simulink model "ex6_dvbs_chain"  (R2022a)
settings: Solver=FixedStepAuto  StartTime=0  StopTime=Tsim  RelTol=1e-3
values from neighbouring files (symbols this model uses):
  Rb = 100e3    (= 100000)    [ex6_parameters.m]
  RS_k = 188    [ex6_parameters.m]
  RS_m = 8    [ex6_parameters.m]
  RS_n = 204    [ex6_parameters.m]
  RS_prim_poly = 'X^8+X^4+X^3+X^2+1'    [ex6_parameters.m]
  VIT_cv1 = 171    [ex6_parameters.m]
  VIT_cv2 = 133    [ex6_parameters.m]
  VIT_K = 7    [ex6_parameters.m]
undefined symbols (not defined in the file or in its folder): rsgenpoly
libraries: commsink2 x2, commblkcod2 x2, commcnvcod2 x2, commsequence2 x2, commblkintrlv2 x2, commrandsrc3 x1, commchan3 x1
settings Model: Creator=root  LastModifiedBy=Filippo
settings SolverCC: AlgebraicLoopSolver=TrustRegion
settings DataIOCC: ReturnWorkspaceOutputs=off
settings DebuggingCC: UnconnectedInputMsg=warning  UnconnectedOutputMsg=warning  UnconnectedLineMsg=warning  SFMachineParentedDataDiag=warning  ArithmeticOperatorsInVariantConditions=warning
settings SFSimCC: SimUseLocalCustomCode=off  CustomCodeUndefinedFunction=UseInterfaceOnly
settings RTWCC: RTWUseLocalCustomCode=off
settings CodeAppCC: StateflowObjectComments=on

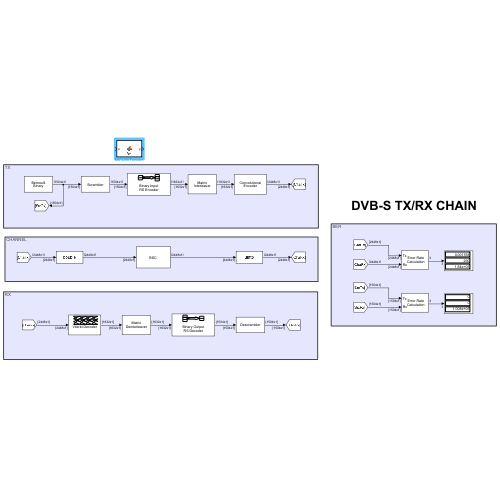
[thumbnail: Simulink's stored preview of the top-level diagram]
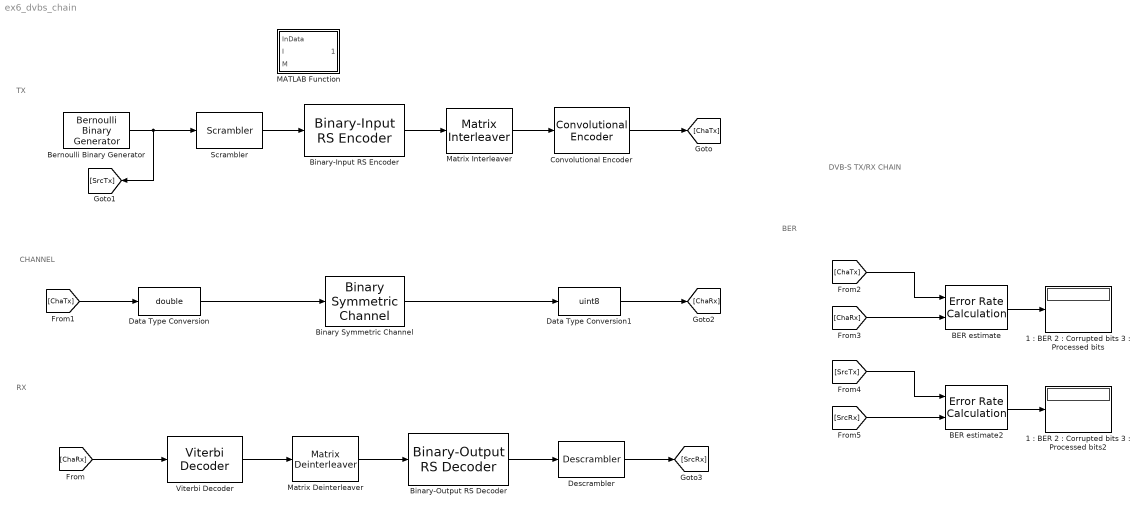
== system ex6_dvbs_chain ==
  note: BER
  note: RX
  note: CHANNEL
  note: TX
  note: DVB-S TX/RX CHAIN
  "1 : BER 2 : Corrupted bits 3 : Processed bits" : Display
  "1 : BER 2 : Corrupted bits 3 : Processed bits2" : Display
  BER estimate : commsink2/Error Rate Calculation  N=0  st_delay=0  cp_mode=Entire frame  subframe=[]  PMode=Port  WsName=ErrorVec  RsMode2=off  stop=off  numErr=100  maxBits=1e6
  BER estimate2 : commsink2/Error Rate Calculation  N=0  st_delay=0  cp_mode=Entire frame  subframe=[]  PMode=Port  WsName=ErrorVec  RsMode2=off  stop=off  numErr=100  maxBits=1e6
  Bernoulli Binary Generator : commrandsrc3/Bernoulli Binary Generator  ProbabilityOfZero=0.5  SeedSource=Auto  Seed=0  SampleTime=1/Rb  SamplesPerFrame=RS_k*RS_m  OutputDataType=uint8  SimulateUsing=Interpreted execution
  Binary Symmetric Channel : commchan3/Binary Symmetric Channel  ErrorProbability=2e-3  ErrorVectorOutputPort=off  OutputDataType=double  OutputDataTypeSL=double  Seed=randi(5000)  SimulateUsing=Code generation
      settings: SourceProductBaseCode=CM
  Binary-Input RS Encoder : commblkcod2/Binary-Input RS Encoder  n=2^RS_m-1  k=2^RS_m-1-(RS_n-RS_k)  specShortening=on  shortenedK=RS_k  specGenPoly=on  genPoly=rsgenpoly(2^RS_m-1, 2^RS_m-1-RS_n+RS_k, RS_prim_poly, [], 'double')  specPrimPoly=on  prPoly=RS_prim_poly  specPuncture=off  punctVec=[ones(2,1); zeros(2,1)]  outDType=Same as input
      settings: SourceProductBaseCode=CM
  Binary-Output RS Decoder : commblkcod2/Binary-Output RS Decoder  n=RS_n  k=RS_k  specShortening=off  shortenedK=RS_k  specGenPoly=on  genPoly=rsgenpoly(2^RS_m-1, 2^RS_m-1-RS_n+RS_k, RS_prim_poly, [], 'double')  specPrimPoly=on  prPoly=RS_prim_poly  specPuncture=off  punctVec=[ones(2,1); zeros(2,1)]  specErasurePort=off  showNumErr=off  outDType=Same as input
      settings: SourceProductBaseCode=CM
  Convolutional Encoder : commcnvcod2/Convolutional Encoder  trellis=poly2trellis(VIT_K, [VIT_cv1 VIT_cv2])  opMode=Truncated (reset every frame)  DelayedResetAction=on  hasIniStPort=off  hasFinStPort=off  usePuncVector=on  punctureVector=VIT_pv  reset=Unused parameter value
      settings: SourceProductBaseCode=CM
  Data Type Conversion : DataTypeConversion  OutDataTypeStr=double  SaturateOnIntegerOverflow=off  RndMeth=Floor
  Data Type Conversion1 : DataTypeConversion  OutDataTypeStr=uint8  SaturateOnIntegerOverflow=off  RndMeth=Floor
  Descrambler : commsequence2/Descrambler  M=2  poly=SCR_poly  iniStaSource=Dialog Parameter  ini_sta=SCR_init  resetViaPort=off
      settings: SourceProductBaseCode=CM
  MATLAB Function : MATLAB Function  TreatAsAtomicUnit=on
  Matrix Deinterleaver : commblkintrlv2/Matrix Deinterleaver  StatePerturbationForJacobian=1.0e-05  Nrows=INT_I  Ncols=INT_M
      settings: SourceProductBaseCode=CM
  Matrix Interleaver : commblkintrlv2/Matrix Interleaver  StatePerturbationForJacobian=1.0e-05  Nrows=INT_I  Ncols=INT_M
      settings: SourceProductBaseCode=CM
  Scrambler : commsequence2/Scrambler  M=2  poly=SCR_poly  iniStaSource=Dialog Parameter  ini_sta=SCR_init  resetViaPort=off
      settings: SourceProductBaseCode=CM
  Viterbi Decoder : commcnvcod2/Viterbi Decoder  trellis=poly2trellis(VIT_K, [VIT_cv1 VIT_cv2])  isPunctured=on  punctureVector=VIT_pv  erasures=off  dectype=Hard decision  nsdecb=4  runSigValErrCheck=off  tbdepth=VIT_td  opmode=Truncated  reset=off  delayedResetAction=off  smWordLength=16  outDataType=Inherit via internal rule
      settings: SourceProductBaseCode=CM
  wires:
  BER estimate/1 -> "1 : BER 2 : Corrupted bits 3 : Processed bits"/1
  Matrix Deinterleaver/1 -> Binary-Output RS Decoder/1
  Bernoulli Binary Generator/1 -> [SrcTx], Scrambler/1
  Binary-Input RS Encoder/1 -> Matrix Interleaver/1
  Scrambler/1 -> Binary-Input RS Encoder/1
  Binary-Output RS Decoder/1 -> Descrambler/1
  Data Type Conversion/1 -> Binary Symmetric Channel/1
  Binary Symmetric Channel/1 -> Data Type Conversion1/1
  [ChaTx] -> Data Type Conversion/1
  Data Type Conversion1/1 -> [ChaRx]
  Descrambler/1 -> [SrcRx]
  [ChaRx] -> BER estimate/2
  [ChaTx] -> BER estimate/1
  [ChaRx] -> Viterbi Decoder/1
  Viterbi Decoder/1 -> Matrix Deinterleaver/1
  Convolutional Encoder/1 -> [ChaTx]
  Matrix Interleaver/1 -> Convolutional Encoder/1
  [SrcTx] -> BER estimate2/1
  [SrcRx] -> BER estimate2/2
  BER estimate2/1 -> "1 : BER 2 : Corrupted bits 3 : Processed bits2"/1

== matlab function ex6_dvbs_chain/MATLAB Function ==
  data: InData input; OutData output; I input; M input

% >> Function for implementing a convolutional interleaver. It requires as the data vector
%    and the number of delay lines (I) and the number of delay cells per block (M). 
function OutData   = CnvIntrlv( InData, I, M )
    Len = length(InData);                                                           % overall I/O buffers length
    OutData = zeros(1,Len);
    ShReg = NaN(I-1,M*(I-1));                                                       % shift register matrix (NaN means the cell is empty)
    InIdx = 1;                                                                      % index over input array
    OutIdx = 1;                                                                     % index over output array
    RwIdx = 0;                                                                      % row index ("0" represents the line with no delay)
    while InIdx <= Len                                                              % loop until all input elements are consumed...
        if RwIdx == 0
            OutData(OutIdx) = InData(InIdx);                                        % output from no-delay line
            OutIdx = OutIdx+1;
        else 
            if ~(isnan(ShReg(RwIdx,M*RwIdx)))
                OutData(OutIdx) = ShReg(RwIdx,M*RwIdx);                             % output from shift-registers
                OutIdx = OutIdx+1;
            end
            for j = M*(RwIdx):-1:2
                ShReg(RwIdx,j) = ShReg(RwIdx,j-1);                                  % update shift-registers (by right-shifting)
            end
            ShReg(RwIdx,1) = InData(InIdx);
        end
        InIdx = InIdx+1;
        
        if RwIdx == I-1
            RwIdx = 0;
        else
            RwIdx = RwIdx+1;
        end
    end
    if RwIdx == 0
        RwIdx = 1;
    end
    while OutIdx <= Len                                                             % loop until all elements still stored in the shift-register has been completely consumed...
        if ~(isnan(ShReg(RwIdx,M*RwIdx)))
            OutData(OutIdx) = ShReg(RwIdx,M*RwIdx);
            OutIdx = OutIdx+1;
        end
        for j = M*(RwIdx):-1:2
            ShReg(RwIdx,j) = ShReg(RwIdx,j-1);
        end
        ShReg(RwIdx,1) = NaN;
        if RwIdx == I-1
            RwIdx = 1;
        else
            RwIdx = RwIdx+1;
        end
    end
end
